simulink model "bracoflc"  (Simulink 10.3)
settings: Solver=ode45  StartTime=0.0  StopTime=10  RelTol=1e-3  AbsTol=1e-6
libraries: fuzblock x1
settings Model: Creator=leize  LastModifiedBy=jhaid  MultithreadedSim=on
settings DataIOCC: SaveOutput=off  SaveTime=off
settings OptimizationCC: BlockReduction=off  BooleanDataType=off  ExpressionDepthLimit=128  LifeSpan=auto
settings DebuggingCC: SaveWithParameterizedLinksMsg=none  SignalResolutionControl=TryResolveAllWithWarning  MultiTaskDSMMsg=warning  MultiTaskCondExecSysMsg=none  FcnCallInpInsideContextMsg=error  StateNameClashWarn=none  SFUnexpectedBacktrackingDiag=error  SFNoUnconditionalDefaultTransitionDiag=error  SFExecutionAtInitializationDiag=warning  ArithmeticOperatorsInVariantConditions=error
settings HardwareCC: ProdBitPerPointer=64  ProdBitPerSizeT=64  ProdBitPerPtrDiffT=64  ProdLargestAtomicFloat=Float  ProdIntDivRoundTo=Zero  ProdEndianess=LittleEndian  ProdWordSize=64  ProdHWDeviceType=Intel->x86-64 (Windows64)  TargetUnknown=on
settings SFSimCC: SimUseLocalCustomCode=on  CustomCodeUndefinedFunction=FilterOut
settings RTWCC: RTWUseLocalCustomCode=on
settings CodeAppCC: StateflowObjectComments=off
settings GRTTargetCC: TargetLangStandard=C99 (ISO)  CombineOutputUpdateFcns=on  GRTInterface=off
settings ConfigComp: CovMetricSettings=dwe  CovSaveCumulativeToWorkspaceVar=off  CovSaveSingleToWorkspaceVar=off  CovExternalEMLEnable=on

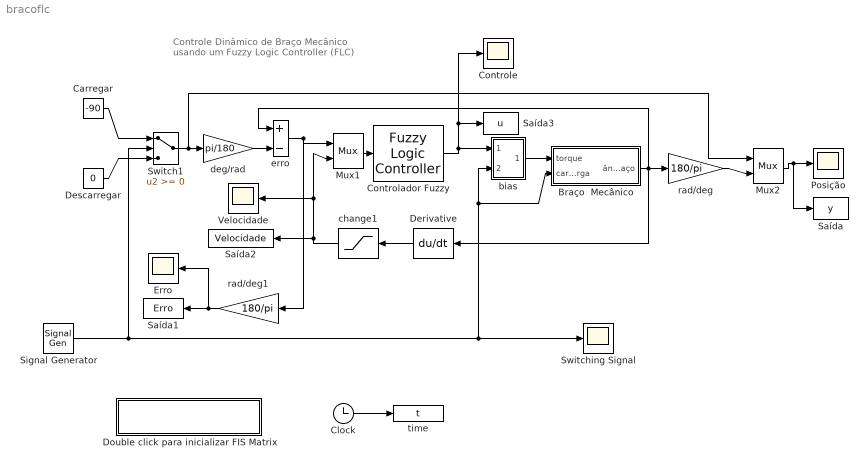
== system bracoflc ==
  note: Controle Dinâmico de Braço Mecânico
      | usando um Fuzzy Logic Controller (FLC)
  " Controlador Fuzzy" : fuzblock/Fuzzy Logic  Controller  FIS='braco.fis'  OutputSampleNumber=101  DataType=double  FuzzifiedInputs=off  RuleFiringStrengths=off  RuleOutputs=off  AggregatedOutputs=off  SimulateUsing=Interpreted execution  OutOfRangeInputValueMessage=warning  NoRuleFiredMessage=warning  EmptyOutputFuzzySetMessage=warning
  Braço  Mecânico : Subsystem  mask{m1=0.5, ml=1, a1=0.75, b1=0.1, g=9.8, xi=|}
      mask xi=|
      | [-1.570796327
      | ; 0]
      mask prompts: m1 "Massa do braço:"; ml "Massa da carga:"; a1 "Comprimento do eixo:"; b1 "Coeficiente de atrito viscoso:"; g "Gravidade:"; xi "Posição Inicial (rad e rad/s):"
      mask help: Braço mecânico
      mask Display: disp('Braço Mecânico')
  Carregar : Constant  Value=-90
  Clock : Clock
  Controle : Scope
  Derivative : Derivative
  Descarregar : Constant  Value=0
  Double click para inicializar FIS Matrix : Subsystem
      settings: OpenFcn=initbraco
      mask Display: disp('Inicializa FisMatrix')
  Erro : Scope
  Mux1 : Mux  Inputs=2
  Mux2 : Mux  Inputs=2
  Posição : Scope
  Saída : ToWorkspace  VariableName=y  SampleTime=-1
  Saída1 : ToWorkspace  VariableName=Erro  SampleTime=-1
  Saída2 : ToWorkspace  VariableName=Velocidade  SampleTime=-1
  Saída3 : ToWorkspace  VariableName=u  SampleTime=-1
  Signal Generator : SignalGenerator  WaveForm=square  Frequency=0.25
  Switch1 : Switch  SaturateOnIntegerOverflow=on  InputSameDT=on
  Switching Signal : Scope
  Velocidade : Scope
  bias : Subsystem  mask{mb=0.5, mc=1, d=0.75, g=9.8}
      mask prompts: mb "Massa do braço mecânico:"; mc "Massa da carga:"; d "Comprimento do eixo:"; g "Gravidade:"
      mask help: Bias
      mask Display: disp('Bias')
  change1 : Saturate  UpperLimit=10  LowerLimit=-10
  deg/rad : Gain  Gain=pi/180  SaturateOnIntegerOverflow=on  OutDataTypeStr=Inherit: Same as input  ParamDataTypeStr=Inherit: Same as input
  erro : Sum  Inputs=+-  InputSameDT=on  SaturateOnIntegerOverflow=on  OutDataTypeStr=Inherit: Same as first input
  rad/deg : Gain  Gain=180/pi  SaturateOnIntegerOverflow=on  OutDataTypeStr=Inherit: Same as input  ParamDataTypeStr=Inherit: Same as input
  rad/deg1 : Gain  Gain=180/pi  SaturateOnIntegerOverflow=on  OutDataTypeStr=Inherit: Same as input  ParamDataTypeStr=Inherit: Same as input
  time : ToWorkspace  VariableName=t
      settings: MaxDataPoints=50000
  wires:
  rad/deg1/1 -> Erro/1, Saída1/1
  Signal Generator/1 -> Switching Signal/1, Braço  Mecânico/2(carga/descarga), bias/2("chaveamento "), Switch1/2
  Clock/1 -> time/1
  change1/1 -> Saída2/1, Mux1/2, Velocidade/1
  Mux2/1 -> Saída/1, Posição/1
  Braço  Mecânico/1(ângulo do braço) -> Derivative/1, erro/1, rad/deg/1
  rad/deg/1 -> Mux2/2
  erro/1 -> rad/deg1/1, Mux1/1
  Derivative/1 -> change1/1
  " Controlador Fuzzy"/1 -> Saída3/1, Controle/1, bias/1(Sinal de controle)
  Mux1/1 -> " Controlador Fuzzy"/1
  Carregar/1 -> Switch1/1
  Descarregar/1 -> Switch1/3
  bias/1(Sinal de Controle com bias) -> Braço  Mecânico/1(torque)
  deg/rad/1 -> erro/2
  Switch1/1 -> deg/rad/1, Mux2/1

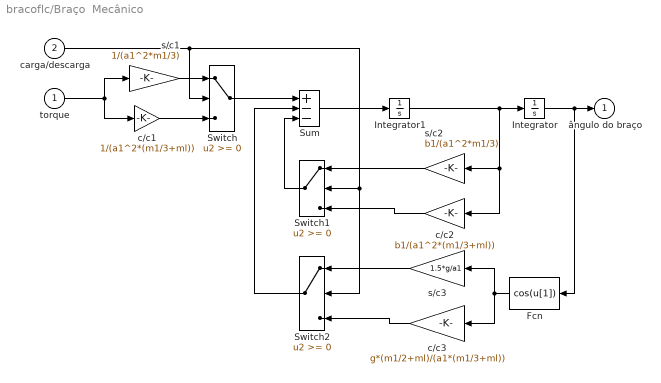
== system bracoflc/Braço  Mecânico ==
  torque : Inport
  carga/descarga : Inport  Port=2
  Fcn : Fcn  Expr=cos(u[1])
  Integrator : Integrator  InitialCondition=xi(1)
  Integrator1 : Integrator  InitialCondition=xi(2)
  Sum : Sum  Inputs=+--  InputSameDT=on  SaturateOnIntegerOverflow=on  OutDataTypeStr=Inherit: Same as first input
  Switch : Switch  SaturateOnIntegerOverflow=on  InputSameDT=on
  Switch1 : Switch  SaturateOnIntegerOverflow=on  InputSameDT=on
  Switch2 : Switch  SaturateOnIntegerOverflow=on  InputSameDT=on
  c/c1 : Gain  Gain=1/(a1^2*(m1/3+ml))  SaturateOnIntegerOverflow=on  OutDataTypeStr=Inherit: Same as input  ParamDataTypeStr=Inherit: Same as input
  c/c2 : Gain  Gain=b1/(a1^2*(m1/3+ml))  SaturateOnIntegerOverflow=on  OutDataTypeStr=Inherit: Same as input  ParamDataTypeStr=Inherit: Same as input
  c/c3 : Gain  Gain=g*(m1/2+ml)/(a1*(m1/3+ml))  SaturateOnIntegerOverflow=on  OutDataTypeStr=Inherit: Same as input  ParamDataTypeStr=Inherit: Same as input
  "s/c1 " : Gain  Gain=1/(a1^2*m1/3)  SaturateOnIntegerOverflow=on  OutDataTypeStr=Inherit: Same as input  ParamDataTypeStr=Inherit: Same as input
  s/c2 : Gain  Gain=b1/(a1^2*m1/3)  SaturateOnIntegerOverflow=on  OutDataTypeStr=Inherit: Same as input  ParamDataTypeStr=Inherit: Same as input
  s/c3 : Gain  Gain=1.5*g/a1  SaturateOnIntegerOverflow=on  OutDataTypeStr=Inherit: Same as input  ParamDataTypeStr=Inherit: Same as input
  ângulo do braço : Outport  InitialOutput=0
  wires:
  Fcn/1 -> c/c3/1, s/c3/1
  c/c2/1 -> Switch1/3
  Switch2/1 -> Sum/2
  c/c3/1 -> Switch2/3
  Integrator1/1 -> s/c2/1, c/c2/1, Integrator/1
  Integrator/1 -> Fcn/1, ângulo do braço/1
  Sum/1 -> Integrator1/1
  "s/c1 "/1 -> Switch/1
  s/c2/1 -> Switch1/1
  s/c3/1 -> Switch2/1
  c/c1/1 -> Switch/3
  Switch1/1 -> Sum/3
  torque/1 -> c/c1/1, "s/c1 "/1
  carga/descarga/1 -> Switch1/2, Switch2/2, Switch/2
  Switch/1 -> Sum/1

== system bracoflc/Double click para inicializar FIS Matrix ==

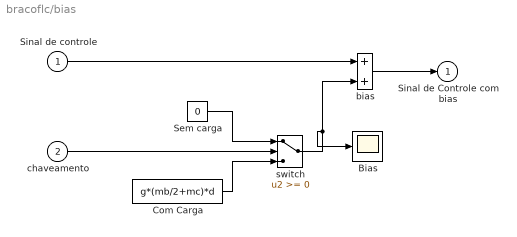
== system bracoflc/bias ==
  Sinal de controle : Inport
  "chaveamento " : Inport  Port=2
  Bias : Scope
  Com Carga : Constant  Value=g*(mb/2+mc)*d
  Sem carga : Constant  Value=0
  bias : Sum  InputSameDT=on  SaturateOnIntegerOverflow=on  OutDataTypeStr=Inherit: Same as first input
  switch : Switch  SaturateOnIntegerOverflow=on  InputSameDT=on
  Sinal de Controle com bias : Outport  InitialOutput=0
  wires:
  bias/1 -> Sinal de Controle com bias/1
  Sinal de controle/1 -> bias/1
  Com Carga/1 -> switch/3
  Sem carga/1 -> switch/1
  "chaveamento "/1 -> switch/2
  switch/1 -> bias/2, Bias/1
